simulink model "TheBigOne"  (R2023b)
settings: Solver=FixedStepAuto  StartTime=0.0  StopTime=800.0  RelTol=1e-3
libraries: simulink x5
(part 2 of 2)

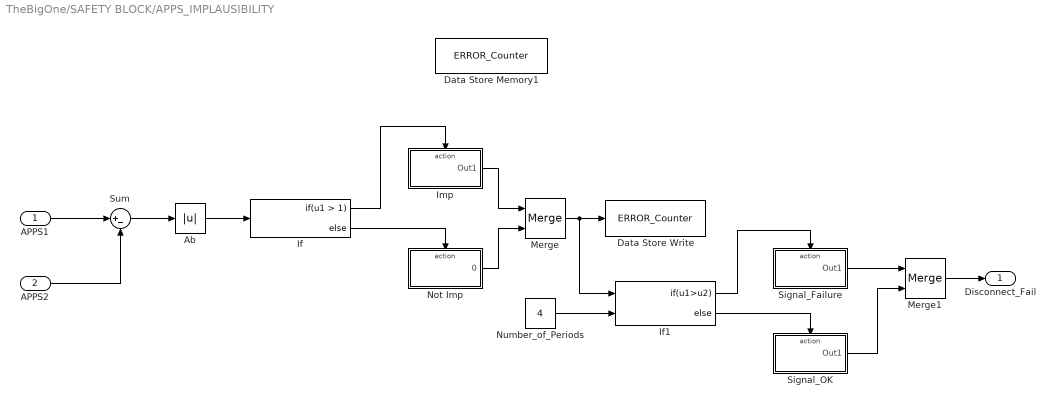
== system TheBigOne/SAFETY BLOCK/APPS_IMPLAUSIBILITY ==
  APPS1 : Inport
  APPS2 : Inport  Port=2
  Ab : Abs  SaturateOnIntegerOverflow=off
  Data Store Memory1 : DataStoreMemory  DataStoreName=ERROR_Counter  ReadBeforeWriteMsg=warning  WriteAfterWriteMsg=warning  WriteAfterReadMsg=warning  ShowAdditionalParam=off
  Data Store Write : DataStoreWrite  DataStoreName=ERROR_Counter  IndexOptions=Index vector (dialog)  Indices=1  OutputSizes=1
  If : If  IfExpression=u1 > 1
  If1 : If  NumInputs=2  IfExpression=u1>u2
  Imp : Subsystem  TreatAsAtomicUnit=on
  Merge : Merge
  Merge1 : Merge
  Not Imp : Subsystem  TreatAsAtomicUnit=on
  Number_of_Periods : Constant  Value=4
  Signal_Failure : Subsystem  TreatAsAtomicUnit=on
  Signal_OK : Subsystem  TreatAsAtomicUnit=on
  Sum : Sum  Inputs=|+-
  Disconnect_Fail : Outport  VectorParamsAs1DForOutWhenUnconnected=off
  wires:
  Number_of_Periods/1 -> If1/2
  Imp/1(Out1) -> Merge/1
  Signal_Failure/1(Out1) -> Merge1/1
  Signal_OK/1(Out1) -> Merge1/2
  Merge1/1 -> Disconnect_Fail/1
  APPS1/1 -> Sum/1
  If/1 -> Imp/Action
  If1/2 -> Signal_OK/Action
  Merge/1 -> Data Store Write/1, If1/1
  If1/1 -> Signal_Failure/Action
  APPS2/1 -> Sum/2
  Ab/1 -> If/1
  If/2 -> Not Imp/Action
  Sum/1 -> Ab/1
  Not Imp/1(0) -> Merge/2

== system TheBigOne/SKIDPAD/RIGIDAXLE ==
  note: TOTAL FAILURE: NO ELIPSE NO INVERTER SPEED
  Throttle_Torque [Nm] : Inport
  Action Port : ActionPort  ActionPortLabel=else
  "Rigid Axle 2024 " : MATLAB Function  TreatAsAtomicUnit=on
  RigidAxle : Constant  Value=4
  Tq_RR_SM4 [Nm] (0,27) : Outport  VectorParamsAs1DForOutWhenUnconnected=off
  Tq_RL_SM4 [Nm] (0,27) : Outport  Port=2  VectorParamsAs1DForOutWhenUnconnected=off
  sensorics_mode : Outport  Port=3
  wires:
  "Rigid Axle 2024 "/1(Motor_Torque_RR) -> Tq_RR_SM4 [Nm] (0,27)/1
  "Rigid Axle 2024 "/2(Motor_Torque_RL) -> Tq_RL_SM4 [Nm] (0,27)/1
  Throttle_Torque [Nm]/1 -> "Rigid Axle 2024 "/1(Throttle_Torque)
  RigidAxle/1 -> sensorics_mode/1

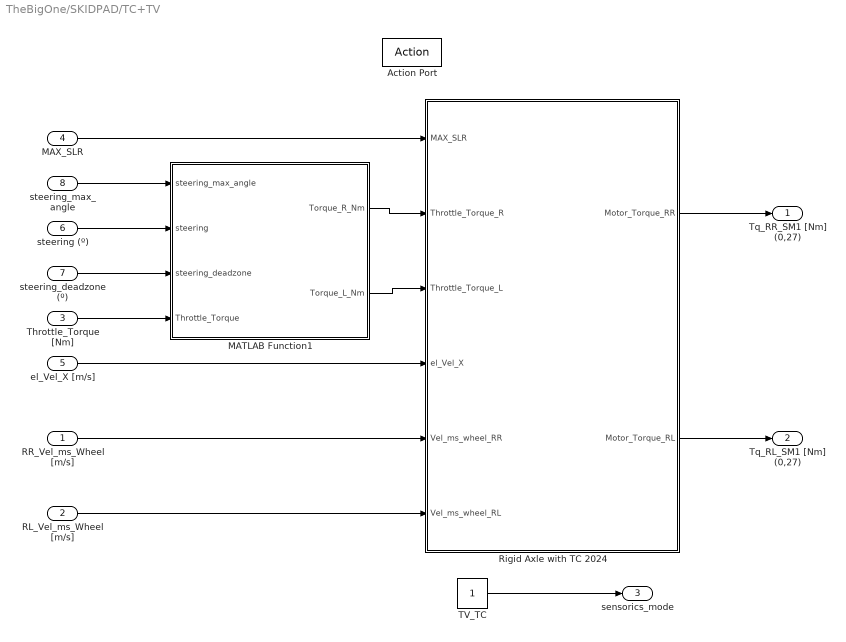
== system TheBigOne/SKIDPAD/TC+TV ==
  RR_Vel_ms_Wheel [m/s] : Inport
  RL_Vel_ms_Wheel [m/s] : Inport  Port=2
  Throttle_Torque [Nm] : Inport  Port=3
  MAX_SLR : Inport  Port=4
  el_Vel_X [m/s] : Inport  Port=5
  steering (º) : Inport  Port=6
  steering_deadzone (º) : Inport  Port=7
  steering_max_angle : Inport  Port=8
  Action Port : ActionPort  ActionPortLabel=if(u1 == 1)
  MATLAB Function1 : MATLAB Function  TreatAsAtomicUnit=on
  "Rigid Axle with TC 2024 " : MATLAB Function  TreatAsAtomicUnit=on
  TV_TC : Constant
  Tq_RR_SM1 [Nm] (0,27) : Outport  VectorParamsAs1DForOutWhenUnconnected=off
  Tq_RL_SM1 [Nm] (0,27) : Outport  Port=2  VectorParamsAs1DForOutWhenUnconnected=off
  sensorics_mode : Outport  Port=3
  wires:
  RR_Vel_ms_Wheel [m/s]/1 -> "Rigid Axle with TC 2024 "/5(Vel_ms_wheel_RR)
  "Rigid Axle with TC 2024 "/1(Motor_Torque_RR) -> Tq_RR_SM1 [Nm] (0,27)/1
  "Rigid Axle with TC 2024 "/2(Motor_Torque_RL) -> Tq_RL_SM1 [Nm] (0,27)/1
  RL_Vel_ms_Wheel [m/s]/1 -> "Rigid Axle with TC 2024 "/6(Vel_ms_wheel_RL)
  Throttle_Torque [Nm]/1 -> MATLAB Function1/4(Throttle_Torque)
  MATLAB Function1/1(Torque_R_Nm) -> "Rigid Axle with TC 2024 "/2(Throttle_Torque_R)
  MAX_SLR/1 -> "Rigid Axle with TC 2024 "/1(MAX_SLR)
  el_Vel_X [m/s]/1 -> "Rigid Axle with TC 2024 "/4(el_Vel_X)
  steering (º)/1 -> MATLAB Function1/2(steering)
  steering_deadzone (º)/1 -> MATLAB Function1/3(steering_deadzone)
  steering_max_angle/1 -> MATLAB Function1/1(steering_max_angle)
  MATLAB Function1/2(Torque_L_Nm) -> "Rigid Axle with TC 2024 "/3(Throttle_Torque_L)
  TV_TC/1 -> sensorics_mode/1

== system TheBigOne/SKIDPAD/TV with TC OFF  ==
  Throttle_Torque [Nm] : Inport
  steering_deadzone : Inport  Port=2
  steering : Inport  Port=3
  steering_max_angle : Inport  Port=4
  Action Port : ActionPort  ActionPortLabel=elseif(u1 <= 3)
  MATLAB Function : MATLAB Function  TreatAsAtomicUnit=on
  SteeringTV : Constant  Value=3
  Tq_RR_SM3 [Nm] (0,27) : Outport  VectorParamsAs1DForOutWhenUnconnected=off
  Tq_RL_SM3 [Nm] (0,27) : Outport  Port=2  VectorParamsAs1DForOutWhenUnconnected=off
  sensorics_mode : Outport  Port=3
  wires:
  Throttle_Torque [Nm]/1 -> MATLAB Function/4(Throttle_Torque)
  steering_deadzone/1 -> MATLAB Function/3(steering_deadzone)
  steering/1 -> MATLAB Function/2(steering)
  steering_max_angle/1 -> MATLAB Function/1(steering_max_angle)
  MATLAB Function/1(Torque_R_Nm) -> Tq_RR_SM3 [Nm] (0,27)/1
  MATLAB Function/2(Torque_L_Nm) -> Tq_RL_SM3 [Nm] (0,27)/1
  SteeringTV/1 -> sensorics_mode/1

== system TheBigOne/TEST_MODE_IN/BYPASS ==
  In1 : Inport
  In2 : Inport  Port=2
  In3 : Inport  Port=3
  In4 : Inport  Port=4
  Action Port : ActionPort  ActionPortLabel=else
  Out1 : Outport  VectorParamsAs1DForOutWhenUnconnected=off
  Out2 : Outport  Port=2  VectorParamsAs1DForOutWhenUnconnected=off
  Out3 : Outport  Port=3  VectorParamsAs1DForOutWhenUnconnected=off
  Out4 : Outport  Port=4  VectorParamsAs1DForOutWhenUnconnected=off
  wires:
  In1/1 -> Out1/1
  In2/1 -> Out2/1
  In3/1 -> Out3/1
  In4/1 -> Out4/1

== system TheBigOne/TEST_MODE_IN/TEST_CONSTANTS ==
  Action Port : ActionPort  ActionPortLabel=if(u1 == 1)
  Constant{,1..3} (4 alike) : Constant  Value=800
  Out1 : Outport  VectorParamsAs1DForOutWhenUnconnected=off
  Out2 : Outport  Port=2  VectorParamsAs1DForOutWhenUnconnected=off
  Out3 : Outport  Port=3  VectorParamsAs1DForOutWhenUnconnected=off
  Out4 : Outport  Port=4  VectorParamsAs1DForOutWhenUnconnected=off
  wires:
  Constant/1 -> Out1/1
  Constant1/1 -> Out2/1
  Constant2/1 -> Out3/1
  Constant3/1 -> Out4/1

== system TheBigOne/Accumulator Power/PowerLimitDetection/LimitReached ==
  Action Port : ActionPort  ActionPortLabel=if(u1 >= 80000)
  Constant : Constant
  "Out " : Outport  VectorParamsAs1DForOutWhenUnconnected=off
  wires:
  Constant/1 -> "Out "/1

== system TheBigOne/Accumulator Power/PowerLimitDetection/OK_OrLatch ==
  IN : Inport
  Action Port : ActionPort  ActionPortLabel=else
  If : If  IfExpression=(u1>0)
  Latched Error : Subsystem  TreatAsAtomicUnit=on
  Merge : Merge
  OK : Subsystem  TreatAsAtomicUnit=on
  Out 1 : Outport  VectorParamsAs1DForOutWhenUnconnected=off
  wires:
  IN/1 -> If/1
  If/1 -> Latched Error/Action
  If/2 -> OK/Action
  Latched Error/1("Out ") -> Merge/1
  OK/1("Out ") -> Merge/2
  Merge/1 -> Out 1/1

== system TheBigOne/ENDURANCE/Velocity cap/If Action Subsystem ==
  Tq_RR : Inport
  Tq_RL : Inport  Port=2
  Action Port : ActionPort  ActionPortLabel=if(u1 > 9)
  Gain : Gain  Gain=0.25
  Gain1 : Gain  Gain=0.25
  TQ_RR : Outport
  TQ_RL : Outport  Port=2
  wires:
  Tq_RL/1 -> Gain1/1
  Gain1/1 -> TQ_RL/1
  Tq_RR/1 -> Gain/1
  Gain/1 -> TQ_RR/1

== system TheBigOne/ENDURANCE/Velocity cap/If Action Subsystem1 ==
  Tq_RR : Inport
  Tq_RL : Inport  Port=2
  Action Port : ActionPort  ActionPortLabel=else
  TQ_RL : Outport
  TQ_RR : Outport  Port=2
  wires:
  Tq_RR/1 -> TQ_RR/1
  Tq_RL/1 -> TQ_RL/1

== system TheBigOne/SAFETY BLOCK/APPS_IMPLAUSIBILITY/Imp ==
  Action Port : ActionPort  ActionPortLabel=if(u1 > 1)
  Add : Sum
  Constant : Constant  OutDataTypeStr=boolean
  Data Store Read : DataStoreRead  DataStoreName=ERROR_Counter  IndexOptions=Index vector (dialog)  Indices=1  OutputSizes=1
  Out1 : Outport  VectorParamsAs1DForOutWhenUnconnected=off
  wires:
  Data Store Read/1 -> Add/1
  Constant/1 -> Add/2
  Add/1 -> Out1/1

== system TheBigOne/SAFETY BLOCK/APPS_IMPLAUSIBILITY/Not Imp ==
  Action Port : ActionPort  ActionPortLabel=else
  Constant : Constant  Value=0  OutDataTypeStr=double
  0 : Outport  VectorParamsAs1DForOutWhenUnconnected=off
  wires:
  Constant/1 -> 0/1  "Boolean"

== system TheBigOne/SAFETY BLOCK/APPS_IMPLAUSIBILITY/Signal_Failure ==
  Action Port : ActionPort  ActionPortLabel=if(u1>u2)
  Constant : Constant
  Out1 : Outport  VectorParamsAs1DForOutWhenUnconnected=off
  wires:
  Constant/1 -> Out1/1

== system TheBigOne/SAFETY BLOCK/APPS_IMPLAUSIBILITY/Signal_OK ==
  Action Port : ActionPort  ActionPortLabel=else
  Constant : Constant  Value=0
  Out1 : Outport  VectorParamsAs1DForOutWhenUnconnected=off
  wires:
  Constant/1 -> Out1/1

== system TheBigOne/Accumulator Power/PowerLimitDetection/OK_OrLatch/Latched Error ==
  Action Port : ActionPort  ActionPortLabel=if((u1>0))
  Constant : Constant
  "Out " : Outport  VectorParamsAs1DForOutWhenUnconnected=off
  wires:
  Constant/1 -> "Out "/1

== system TheBigOne/Accumulator Power/PowerLimitDetection/OK_OrLatch/OK ==
  Action Port : ActionPort  ActionPortLabel=else
  Constant : Constant  Value=0
  "Out " : Outport  VectorParamsAs1DForOutWhenUnconnected=off
  wires:
  Constant/1 -> "Out "/1

== matlab function TheBigOne/Brake_Light ==
  data: BP input; RM input; BL output; PS input; BL_threshold input
function BL = Brake_Light(BP, RM, PS, BL_threshold)
% PS = 0 -> braking
% PS = 1 -> lift
% PS = 2 -> accelerating
% BL_threshold -> BrakePedal percentage to activate BrakeLight
    if ((RM == 5 && PS == 0) || (BP > BL_threshold))
        BL = 1;
        return;
    else
        BL = 0;
        return;
    end
end

== matlab function TheBigOne/Safety ==
  data: Tq_R input; Tq_OK input; Tq_L input; Torque_R output; Torque_L output; W_mot_RR input; W_mot_RL input
function [Torque_R,Torque_L]  = Safety(Tq_R, Tq_OK, Tq_L, W_mot_RR, W_mot_RL)
    if Tq_OK == 1
        Torque_R = Tq_R;
        Torque_L = Tq_L;
        return;
    else
        Torque_R = 0;
        Torque_L = 0;
        return;
    end
end

== matlab function TheBigOne/ACCELERATION/RIGIDAXLE/Rigid Axle 2024  ==
  data: Throttle_Torque input; Motor_Torque_RR output; Motor_Torque_RL output
function [Motor_Torque_RR, Motor_Torque_RL] = RigidAxle_2024(Throttle_Torque)
    
    Motor_Torque_RR = Throttle_Torque;
    Motor_Torque_RL = Throttle_Torque;

end

== matlab function TheBigOne/ACCELERATION/RIGIDAXLE WITH TC/Rigid Axle with TC 2024  ==
  data: MAX_SLR input; Throttle_Torque input; Motor_Torque_RR output; Motor_Torque_RL output; el_Vel_X input; Max_Vel_ms_Wheel input
function [Motor_Torque_RR, Motor_Torque_RL] = RigidAxle_TC_2024(MAX_SLR, Throttle_Torque, el_Vel_X, Max_Vel_ms_Wheel)    
    persistent correction
    if isempty(correction)
        correction = 0;
    end
if (el_Vel_X < 0.5 || Max_Vel_ms_Wheel < 0.5)
    correction = 0;
    Motor_Torque_RR = Throttle_Torque;
    Motor_Torque_RL = Throttle_Torque;
    return;
else

% SLIP RATIO CALCULATIONS
    % calculate slip ratio
    if(el_Vel_X == 0 ||Max_Vel_ms_Wheel == 0)
        SLR = 1;
    else
    SLR = (Max_Vel_ms_Wheel / el_Vel_X);
    end
% CHECK FOR EXCESIVE SLIPPING
    % SLIP RATIO LESSER THAN MAXIMUM SLIP RATIO => apply max torque times throttle factor
        if(SLR < MAX_SLR)
            Motor_Torque_RR = Throttle_Torque; 
            Motor_Torque_RL = Throttle_Torque;
            correction = 0; %set correction to 0 as tyre is not slipping
            return;
        else
        % TYRE SLIPPING => TC INTERVENES
            % LOOK FOR THE PREVIOUS CORRECTION [Nm]
            if (correction == 0) % NOT SLIPPING PREVIOUSLY
                correction = 1; % [INTERVAL TO BE DETERMINED] set the correction to the torque we want to substract
                Motor_Torque_RR = Throttle_Torque - (1/33*correction^2+1/33*correction); % substract the correction from the torque to apply
                Motor_Torque_RL = Throttle_Torque - (1/33*correction^2+1/33*correction);
                return;
            else % TYRE SLIPPING PREVIOUSLY
                correction = correction + 1; % [INTERVAL TO BE DETERMINED] set the correction to the torque we want to substract + previous corrections
                Motor_Torque_RR = Throttle_Torque - (1/33*correction^2+1/33*correction); % substract the correction from the torque to apply
                Motor_Torque_RL = Throttle_Torque - (1/33*correction^2+1/33*correction);
                return;
            end
        end
end
end

== matlab function TheBigOne/ENDURANCE/RIGIDAXLE WITH TC/Rigid Axle with TC 2024  ==
  data: MAX_SLR input; Throttle_Torque input; Motor_Torque_RR output; Motor_Torque_RL output; el_Vel_X input; Max_Vel_ms_Wheel input
function [Motor_Torque_RR, Motor_Torque_RL] = RigidAxle_TC_2024(MAX_SLR, Throttle_Torque, el_Vel_X, Max_Vel_ms_Wheel)    
    persistent correction
    if isempty(correction)
        correction = 0;
    end
if (el_Vel_X < 0.5 || Max_Vel_ms_Wheel < 0.5)
    Motor_Torque_RR = Throttle_Torque;
    Motor_Torque_RL = Throttle_Torque;
    return;
else

% SLIP RATIO CALCULATIONS
    % calculate slip ratio
    if(el_Vel_X == 0 ||Max_Vel_ms_Wheel == 0)
        SLR = 1;
    else
    SLR = (Max_Vel_ms_Wheel / el_Vel_X);
    end
% CHECK FOR EXCESIVE SLIPPING
    % SLIP RATIO LESSER THAN MAXIMUM SLIP RATIO => apply max torque times throttle factor
        if(SLR < MAX_SLR)
            Motor_Torque_RR = Throttle_Torque; 
            Motor_Torque_RL = Throttle_Torque;
            correction = 0; %set correction to 0 as tyre is not slipping
            return;
        else
        % TYRE SLIPPING => TC INTERVENES
            % LOOK FOR THE PREVIOUS CORRECTION [Nm]
            if (correction == 0) % NOT SLIPPING PREVIOUSLY
                correction = 1; % [INTERVAL TO BE DETERMINED] set the correction to the torque we want to substract
                Motor_Torque_RR = Throttle_Torque - (1/33*correction^2+1/33*correction); % substract the correction from the torque to apply
                Motor_Torque_RL = Throttle_Torque - (1/33*correction^2+1/33*correction);
                return;
            else % TYRE SLIPPING PREVIOUSLY
                correction = correction + 1; % [INTERVAL TO BE DETERMINED] set the correction to the torque we want to substract + previous corrections
                Motor_Torque_RR = Throttle_Torque - (1/33*correction^2+1/33*correction); % substract the correction from the torque to apply
                Motor_Torque_RL = Throttle_Torque - (1/33*correction^2+1/33*correction);
                return;
            end
        end
end
end

== matlab function TheBigOne/ENDURANCE/TC+TV/TC 2024 ==
  data: MAX_SLR input; Throttle_Torque_R input; Throttle_Torque_L input; Motor_Torque_RR output; Motor_Torque_RL output; el_Vel_X input; Vel_ms_wheel_RR input; Vel_ms_wheel_RL input
function [Motor_Torque_RR, Motor_Torque_RL] = TC_2024(MAX_SLR,Throttle_Torque_R, Throttle_Torque_L, el_Vel_X, Vel_ms_wheel_RR, Vel_ms_wheel_RL)
    persistent correction
    if isempty(correction)
        correction = 0;
    end
if (el_Vel_X < 0.5 || Vel_ms_wheel_RR < 0.5 || Vel_ms_wheel_RL < 0.5)
    Motor_Torque_RR = Throttle_Torque_R;
    Motor_Torque_RL = Throttle_Torque_L;
    return;
else

% SLIP RATIO CALCULATIONS
    % calculate slip ratio
    if(el_Vel_X == 0 || Vel_ms_wheel_RR == 0)
        SLR_RR = 1;
    else
    SLR_RR = (Vel_ms_wheel_RR / el_Vel_X);
    end
    if(el_Vel_X == 0 || Vel_ms_wheel_RL == 0)
        SLR_RL = 1;
    else
    SLR_RL = (Vel_ms_wheel_RL / el_Vel_X);
    end


% SLIP RATIO CALCULATIONS
    % calculate slip ratio
    SLR = max(SLR_RR, SLR_RL);

% CHECK FOR EXCESIVE SLIPPING
    % SLIP RATIO LESSER THAN MAXIMUM SLIP RATIO => apply max torque times throttle factor
        if(SLR < MAX_SLR)
            Motor_Torque_RR = Throttle_Torque_R; 
            Motor_Torque_RL = Throttle_Torque_L;
            correction = 0; %set correction to 0 as tyre is not slipping
            return;
        else
        % TYRE SLIPPING => TC INTERVENES
            % LOOK FOR THE PREVIOUS CORRECTION [Nm]
            if (correction == 0) % NOT SLIPPING PREVIOUSLY
                correction = 1; % [INTERVAL TO BE DETERMINED] set the correction to the torque we want to substract
                Motor_Torque_RR = Throttle_Torque_R - (1/33*correction^2+1/33*correction); % substract the correction from the torque to apply
                Motor_Torque_RL = Throttle_Torque_L - (1/33*correction^2+1/33*correction);
                return;
            else % TYRE SLIPPING PREVIOUSLY
                correction = correction + 1; % [INTERVAL TO BE DETERMINED] set the correction to the torque we want to substract + previous corrections
                Motor_Torque_RR = Throttle_Torque_R - (1/33*correction^2+1/33*correction); % substract the correction from the torque to apply
                Motor_Torque_RL = Throttle_Torque_L - (1/33*correction^2+1/33*correction);
                return;
            end
        end
end
end

== matlab function TheBigOne/ACCELERATION/Torque demanded by the driver ==
  data: Throttle_Torque output; AP input; pedal_sat_down input; pedal_sat_up input; max_torque input
function Throttle_Torque  = TT(AP, pedal_sat_down, pedal_sat_up, max_torque)
    if AP <= pedal_sat_down %establish the lower deadzone for the throttle pedal
        Throttle_Response = 0;

    elseif AP >= pedal_sat_up %establish the higher deadzone for the throttle pedal
        Throttle_Response = 1;

    else
        Throttle_Response = ((AP - pedal_sat_down) / (pedal_sat_up - pedal_sat_down)); %evaluate for given input
    end
    Throttle_Torque = Throttle_Response * max_torque; % set torque to max output times pedal factor
end

== matlab function TheBigOne/InverterL_Temp_Limitation ==
  data: Current_in input; Aggressive_Factor input; Max_Temp input; Current_out output; Tolerance input; Inv_Temp input; Change_Factor input
function Current_out = Inv_Temp(Current_in, Aggressive_Factor, Max_Temp, Tolerance, Inv_Temp, Change_Factor)
%% Initializing internal variables
% If they have not been defined yet, initiate them

    % Last_Temp (ºC) -> Inv_Temp of the last iteration
    persistent Last_Temp
    if isempty(Last_Temp)
        Last_Temp = 0;
    end

    % Aggressive Factor Value (%) -> Factor of Current reduction. Changes
    % every iteration due to counters, but can be reset if the Inv_Temp is
    % acceptable
    persistent AF_Value
    if isempty(AF_Value)
        AF_Value = Aggressive_Factor;
    end

    % Times_Incremented -> Counter of the Temp_Change higher than Tolerance
    persistent Times_Incremented
    if isempty(Times_Incremented)
        Times_Incremented = 1;
    end

    % Times_Decremented -> Counter of the Temp_Change lower than -Tolerance
    persistent Times_Decremented
    if isempty(Times_Decremented)
        Times_Decremented = 1;
    end

%% Derivative
    % Compute the Temperature difference between the last temp and the
    % actual one
Temp_Change = Inv_Temp - Last_Temp;

%% Temperature Control Logic
    
    if (Temp_Change > Tolerance)
        % Temperature is increasing beyond Tolerance, limit the Current
        % more aggressively to reduce the Inv_Temp
        New_Current = Current_in * (1 - (AF_Value * Temp_Change / 100));
        % Increase the Aggresive Factor for the next iteration and sum 1 to
        % the Increment counter
        AF_Value = AF_Value + (Change_Factor * Times_Incremented);
        Times_Incremented = Times_Incremented + 1;
        Times_Decremented = 1;

    elseif (Temp_Change < -Tolerance)
        % Temperature is cooling down beyond Tolerance, allow to normalize
        % the Current (then the temperature rises)
        New_Current = Current_in * (1 - (AF_Value * Temp_Change / 100));
        % Decrease the Aggressive Factor for the next iteration and sum 1
        % to the Decrement counter
        AF_Value = AF_Value - (Change_Factor * Times_Decremented);
        Times_Incremented = 1;
        Times_Decremented = Times_Decremented + 1;

    else
        % Temperature is stable (within Tolerance), gradually reduce Current
        New_Current = Current_in * (1 - AF_Value / 10);
        % Reset both counters
        Times_Incremented = 1;
        Times_Decremented = 1;

    end
%% Compare the Actual Current with the New Current

    if (((New_Current > Current_in) && (Current_in >= 0)) || ((New_Current < Current_in) && (Current_in < 0)))
        % Ensure the New_Current does not exceed the input current when accelerating
        % If regen, then the New_Current cannot be lower than the Current_in, it
        % has to be higher (they are both negative)
        New_Current = Current_in;

    elseif (sign(New_Current) ~= sign(Current_in))
        % If it was demanding a positive current, but New_Current is
        % negative, just output 0 (so we do not regenerate when we don't
        % want). Same for the inverse case
        New_Current = 0;
        
    end

%% Output values

    if (Inv_Temp > Max_Temp)
        % If the Inv_Temp is higher than the Maximum_Temp selected, limit
        % the Current with the calculated one
        Current_out = New_Current;

    else
        % If the Inv_Temp is acceptable, maintain the current demanded and
        % do not apply the calculated Aggresive Factor Value
        Current_out = Current_in;
        AF_Value = Aggressive_Factor;

    end
% Update the last known Temperature
Last_Temp = Inv_Temp;
end

== matlab function TheBigOne/ENDURANCE/Torque/state ==
  data: AP input; AP_sat_down input; state output; AP_sat_mid input
function state = Pedal_State(AP, AP_sat_down, AP_sat_mid)
% state = 0 -> braking
% state = 1 -> lift
% state = 2 -> accelerating
state = 1;
if AP < AP_sat_down
    state = 0;
    return;
end
if AP >= AP_sat_down && AP <= AP_sat_mid
    state = 1;
    return;
end
if AP > AP_sat_mid
    state = 2;
    return;
end
end

== matlab function TheBigOne/AUTOX1/TC+TV/Rigid Axle with TC 2024  ==
  data: MAX_SLR input; Throttle_Torque_R input; Throttle_Torque_L input; Motor_Torque_RR output; Motor_Torque_RL output; el_Vel_X input; Vel_ms_wheel_RR input; Vel_ms_wheel_RL input
function [Motor_Torque_RR, Motor_Torque_RL] = TC_2024(MAX_SLR,Throttle_Torque_R, Throttle_Torque_L, el_Vel_X, Vel_ms_wheel_RR, Vel_ms_wheel_RL)
    persistent correction
    if isempty(correction)
        correction = 0;
    end
if (el_Vel_X < 0.5 || Vel_ms_wheel_RR < 0.5 || Vel_ms_wheel_RL < 0.5)
    correction = 0;
    Motor_Torque_RR = Throttle_Torque_R;
    Motor_Torque_RL = Throttle_Torque_L;
    return;
else
    
% SLIP RATIO CALCULATIONS
    % calculate slip ratio
    if(el_Vel_X == 0 || Vel_ms_wheel_RR == 0)
        SLR_RR = 1;
    else
    SLR_RR = (Vel_ms_wheel_RR / el_Vel_X);
    end
    if(el_Vel_X == 0 || Vel_ms_wheel_RL == 0)
        SLR_RL = 1;
    else
    SLR_RL = (Vel_ms_wheel_RL / el_Vel_X);
    end


% SLIP RATIO CALCULATIONS
    % calculate slip ratio
    SLR = max(SLR_RR, SLR_RL);

% CHECK FOR EXCESIVE SLIPPING
    % SLIP RATIO LESSER THAN MAXIMUM SLIP RATIO => apply max torque times throttle factor
        if(SLR < MAX_SLR)
            Motor_Torque_RR = Throttle_Torque_R; 
            Motor_Torque_RL = Throttle_Torque_L;
            correction = 0; %set correction to 0 as tyre is not slipping
            return;
        else
        % TYRE SLIPPING => TC INTERVENES
            % LOOK FOR THE PREVIOUS CORRECTION [Nm]
            if (correction == 0) % NOT SLIPPING PREVIOUSLY
                correction = 1; % [INTERVAL TO BE DETERMINED] set the correction to the torque we want to substract
                Motor_Torque_RR = Throttle_Torque_R - (1/33*correction^2+1/33*correction); % substract the correction from the torque to apply
                Motor_Torque_RL = Throttle_Torque_L - (1/33*correction^2+1/33*correction);
                return;
            else % TYRE SLIPPING PREVIOUSLY
                correction = correction + 1; % [INTERVAL TO BE DETERMINED] set the correction to the torque we want to substract + previous corrections
                Motor_Torque_RR = Throttle_Torque_R - (1/33*correction^2+1/33*correction); % substract the correction from the torque to apply
                Motor_Torque_RL = Throttle_Torque_L - (1/33*correction^2+1/33*correction);
                return;
            end
        end
end
end

== matlab function TheBigOne/SKIDPAD/TV with TC OFF /MATLAB Function ==
  data: steering_max_angle input; Torque_R_Nm output; Torque_L_Nm output; steering input; steering_deadzone input; Throttle_Torque input
function [Torque_R_Nm, Torque_L_Nm] = TV(steering_max_angle, steering, steering_deadzone, Throttle_Torque)

if abs(steering) <= steering_deadzone % add steering deadzone (º)
    Torque_L_Nm = Throttle_Torque;
    Torque_R_Nm = Throttle_Torque;
    return;
end
d = (abs(steering) - steering_deadzone)/(steering_max_angle - steering_deadzone) * Throttle_Torque; %evaluate delta torque for given steering angle
if d > Throttle_Torque
     d = Throttle_Torque; %force torque to be positive to avoid balance issues
end
if steering < -steering_deadzone %if steering left, apply full torque to the emotor on the outside
    Torque_L_Nm = Throttle_Torque-d;
    Torque_R_Nm = Throttle_Torque;
    return;
else
%opposite case
Torque_L_Nm = Throttle_Torque;
Torque_R_Nm = Throttle_Torque-d;
return;
end
end

== matlab function TheBigOne/WORKSHOP/Torque demanded by the driver ==
  data: Throttle_Torque output; AP input; pedal_sat_down input; pedal_sat_up input; max_torque input; max_wheel_w input
function Throttle_Torque  = TT(AP, pedal_sat_down, pedal_sat_up, max_torque, max_wheel_w)
max_torque = max_torque / 9; % Max Tq = 3Nm
    if AP <= pedal_sat_down || max_wheel_w > 5 % establish the lower deadzone for the throttle pedal
        Throttle_Response = 0;

    elseif AP >= pedal_sat_up % establish the higher deadzone for the throttle pedal
        Throttle_Response = 1;

    else
        Throttle_Response = ((AP - pedal_sat_down) / (pedal_sat_up - pedal_sat_down)); %evaluate for given input
    end
    Throttle_Torque = Throttle_Response * max_torque; % set torque to max output times pedal factor
end

== matlab function TheBigOne/InverterR_Temp_Limitation ==
  data: Current_in input; Aggressive_Factor input; Max_Temp input; Current_out output; Tolerance input; Inv_Temp input; Change_Factor input
function Current_out = Inv_Temp(Current_in, Aggressive_Factor, Max_Temp, Tolerance, Inv_Temp, Change_Factor)
%% Initializing internal variables
% If they have not been defined yet, initiate them

    % Last_Temp (ºC) -> Inv_Temp of the last iteration
    persistent Last_Temp
    if isempty(Last_Temp)
        Last_Temp = 0;
    end

    % Aggressive Factor Value (%) -> Factor of Current reduction. Changes
    % every iteration due to counters, but can be reset if the Inv_Temp is
    % acceptable
    persistent AF_Value
    if isempty(AF_Value)
        AF_Value = Aggressive_Factor;
    end

    % Times_Incremented -> Counter of the Temp_Change higher than Tolerance
    persistent Times_Incremented
    if isempty(Times_Incremented)
        Times_Incremented = 1;
    end

    % Times_Decremented -> Counter of the Temp_Change lower than -Tolerance
    persistent Times_Decremented
    if isempty(Times_Decremented)
        Times_Decremented = 1;
    end

%% Derivative
    % Compute the Temperature difference between the last temp and the
    % actual one
Temp_Change = Inv_Temp - Last_Temp;

%% Temperature Control Logic
    
    if (Temp_Change > Tolerance)
        % Temperature is increasing beyond Tolerance, limit the Current
        % more aggressively to reduce the Inv_Temp
        New_Current = Current_in * (1 - (AF_Value * Temp_Change / 100));
        % Increase the Aggresive Factor for the next iteration and sum 1 to
        % the Increment counter
        AF_Value = AF_Value + (Change_Factor * Times_Incremented);
        Times_Incremented = Times_Incremented + 1;
        Times_Decremented = 1;

    elseif (Temp_Change < -Tolerance)
        % Temperature is cooling down beyond Tolerance, allow to normalize
        % the Current (then the temperature rises)
        New_Current = Current_in * (1 - (AF_Value * Temp_Change / 100));
        % Decrease the Aggressive Factor for the next iteration and sum 1
        % to the Decrement counter
        AF_Value = AF_Value - (Change_Factor * Times_Decremented);
        Times_Incremented = 1;
        Times_Decremented = Times_Decremented + 1;

    else
        % Temperature is stable (within Tolerance), gradually reduce Current
        New_Current = Current_in * (1 - AF_Value / 10);
        % Reset both counters
        Times_Incremented = 1;
        Times_Decremented = 1;

    end
%% Compare the Actual Current with the New Current

    if (((New_Current > Current_in) && (Current_in >= 0)) || ((New_Current < Current_in) && (Current_in < 0)))
        % Ensure the New_Current does not exceed the input current when accelerating
        % If regen, then the New_Current cannot be lower than the Current_in, it
        % has to be higher (they are both negative)
        New_Current = Current_in;

    elseif (sign(New_Current) ~= sign(Current_in))
        % If it was demanding a positive current, but New_Current is
        % negative, just output 0 (so we do not regenerate when we don't
        % want). Same for the inverse case
        New_Current = 0;
        
    end

%% Output values

    if (Inv_Temp > Max_Temp)
        % If the Inv_Temp is higher than the Maximum_Temp selected, limit
        % the Current with the calculated one
        Current_out = New_Current;

    else
        % If the Inv_Temp is acceptable, maintain the current demanded and
        % do not apply the calculated Aggresive Factor Value
        Current_out = Current_in;
        AF_Value = Aggressive_Factor;

    end
% Update the last known Temperature
Last_Temp = Inv_Temp;
end

== matlab function TheBigOne/ENDURANCE/Torque/enable regen ==
  data: regen_en output; SOC input; max_SOC input; current input; voltage input; W_RR input; W_RL input; max_regen_torque_RR output; max_regen_torque_RL output
function [regen_en, max_regen_torque_RR, max_regen_torque_RL] = regen(SOC, max_SOC, current, voltage, W_RR, W_RL)
    max_regen_torque_RR = 0;
    max_regen_torque_RL = 0;
    regen_en = 0;
    if SOC < max_SOC && min(W_RR, W_RL) > 33 %If W is lower (< 2.4 km/h), do not regen to avoid going backwards
        regen_en = 1;
    end
    if SOC >= max_SOC
        regen_en = 0;
    end
    if regen_en == 1
        max_regen_torque_RR = min(current*voltage/W_RR, 27);
        max_regen_torque_RL = min(current*voltage/W_RL, 27);
    end
end

== matlab function TheBigOne/ENDURANCE/Torque/Torque demanded by the driver ==
  data: max_regen_torque input; regen_en input; state input; AP input; AP_sat_down input; AP_sat_mid input; tq_RR output; tq_RL output; max_torque input
function [tq_RR, tq_RL] = torque(max_regen_torque, regen_en, state, AP, AP_sat_down, AP_sat_mid, max_torque)
% state = 0 -> braking
% state = 1 -> lift
% state = 2 -> accelerating
    tq_RR = 0;
    tq_RL = 0;
    if state == 0
        if regen_en == 1
        tq_RR = AP * (max_regen_torque/AP_sat_down) - max_regen_torque;
        tq_RL = tq_RR;
        else
            tq_RR = 0;
            tq_RL = 0;
        end
    end
    if state == 1
        tq_RR = 0;
        tq_RL = 0;
    end
    if state == 2
        tq_RR = max_torque * ((AP-AP_sat_mid) / (1 - AP_sat_mid));
        tq_RL = tq_RR;
    end
end

== matlab function TheBigOne/AUTOX1/RIGIDAXLE/Rigid Axle 2024  ==
  data: Throttle_Torque input; Motor_Torque_RR output; Motor_Torque_RL output
function [Motor_Torque_RR, Motor_Torque_RL] = RigidAxle_2024(Throttle_Torque)
    
    Motor_Torque_RR = Throttle_Torque;
    Motor_Torque_RL = Throttle_Torque;

end

== matlab function TheBigOne/ENDURANCE/RIGIDAXLE/Rigid Axle 2024  ==
  data: Throttle_Torque input; Motor_Torque_RR output; Motor_Torque_RL output
function [Motor_Torque_RR, Motor_Torque_RL] = RigidAxle_2024(Throttle_Torque)
    
    Motor_Torque_RR = Throttle_Torque;
    Motor_Torque_RL = Throttle_Torque;

end

== matlab function TheBigOne/MotorL_Temp_Limitation ==
  data: Current_in input; Aggressive_Factor input; Max_Temp input; Current_out output; Tolerance input; Mot_Temp input; Change_Factor input
function Current_out = Mot_Temp(Current_in, Aggressive_Factor, Max_Temp, Tolerance, Mot_Temp, Change_Factor)
%% Initializing internal variables
% If they have not been defined yet, initiate them

    % Last_Temp (ºC) -> Mot_Temp of the last iteration
    persistent Last_Temp
    if isempty(Last_Temp)
        Last_Temp = 0;
    end

    % Aggressive Factor Value (%) -> Factor of Current reduction. Changes
    % every iteration due to counters, but can be reset if the Mot_Temp is
    % acceptable
    persistent AF_Value
    if isempty(AF_Value)
        AF_Value = Aggressive_Factor;
    end

    % Times_Incremented -> Counter of the Temp_Change higher than Tolerance
    persistent Times_Incremented
    if isempty(Times_Incremented)
        Times_Incremented = 1;
    end

    % Times_Decremented -> Counter of the Temp_Change lower than -Tolerance
    persistent Times_Decremented
    if isempty(Times_Decremented)
        Times_Decremented = 1;
    end

%% Derivative
    % Compute the Temperature difference between the last temp and the
    % actual one
Temp_Change = Mot_Temp - Last_Temp;

%% Temperature Control Logic
    
    if (Temp_Change > Tolerance)
        % Temperature is increasing beyond Tolerance, limit the Current
        % more aggressively to reduce the Mot_Temp
        New_Current = Current_in * (1 - (AF_Value * Temp_Change / 100));
        % Increase the Aggresive Factor for the next iteration and sum 1 to
        % the Increment counter
        AF_Value = AF_Value + (Change_Factor * Times_Incremented);
        Times_Incremented = Times_Incremented + 1;
        Times_Decremented = 1;

    elseif (Temp_Change < -Tolerance)
        % Temperature is cooling down beyond Tolerance, allow to normalize
        % the Current (then the temperature rises)
        New_Current = Current_in * (1 - (AF_Value * Temp_Change / 100));
        % Decrease the Aggressive Factor for the next iteration and sum 1
        % to the Decrement counter
        AF_Value = AF_Value - (Change_Factor * Times_Decremented);
        Times_Incremented = 1;
        Times_Decremented = Times_Decremented + 1;

    else
        % Temperature is stable (within Tolerance), gradually reduce Current
        New_Current = Current_in * (1 - AF_Value / 10);
        % Reset both counters
        Times_Incremented = 1;
        Times_Decremented = 1;

    end
%% Compare the Actual Current with the New Current

    if (((New_Current > Current_in) && (Current_in >= 0)) || ((New_Current < Current_in) && (Current_in < 0)))
        % Ensure the New_Current does not exceed the input current when accelerating
        % If regen, then the New_Current cannot be lower than the Current_in, it
        % has to be higher (they are both negative)
        New_Current = Current_in;

    elseif (sign(New_Current) ~= sign(Current_in))
        % If it was demanding a positive current, but New_Current is
        % negative, just output 0 (so we do not regenerate when we don't
        % want). Same for the inverse case
        New_Current = 0;
        
    end

%% Output values

    if (Mot_Temp > Max_Temp)
        % If the Mot_Temp is higher than the Maximum_Temp selected, limit
        % the Current with the calculated one
        Current_out = New_Current;

    else
        % If the Mot_Temp is acceptable, maintain the current demanded and
        % do not apply the calculated Aggresive Factor Value
        Current_out = Current_in;
        AF_Value = Aggressive_Factor;

    end
% Update the last known Temperature
Last_Temp = Mot_Temp;
end

== matlab function TheBigOne/SKIDPAD/RIGIDAXLE/Rigid Axle 2024  ==
  data: Throttle_Torque input; Motor_Torque_RR output; Motor_Torque_RL output
function [Motor_Torque_RR, Motor_Torque_RL] = RigidAxle_2024(Throttle_Torque)
    
    Motor_Torque_RR = Throttle_Torque;
    Motor_Torque_RL = Throttle_Torque;

end

== matlab function TheBigOne/MotorR_Temp_Limitation ==
  data: Current_in input; Aggressive_Factor input; Max_Temp input; Current_out output; Tolerance input; Mot_Temp input; Change_Factor input
function Current_out = Mot_Temp(Current_in, Aggressive_Factor, Max_Temp, Tolerance, Mot_Temp, Change_Factor)
%% Initializing internal variables
% If they have not been defined yet, initiate them

    % Last_Temp (ºC) -> Mot_Temp of the last iteration
    persistent Last_Temp
    if isempty(Last_Temp)
        Last_Temp = 0;
    end

    % Aggressive Factor Value (%) -> Factor of Current reduction. Changes
    % every iteration due to counters, but can be reset if the Mot_Temp is
    % acceptable
    persistent AF_Value
    if isempty(AF_Value)
        AF_Value = Aggressive_Factor;
    end

    % Times_Incremented -> Counter of the Temp_Change higher than Tolerance
    persistent Times_Incremented
    if isempty(Times_Incremented)
        Times_Incremented = 1;
    end

    % Times_Decremented -> Counter of the Temp_Change lower than -Tolerance
    persistent Times_Decremented
    if isempty(Times_Decremented)
        Times_Decremented = 1;
    end

%% Derivative
    % Compute the Temperature difference between the last temp and the
    % actual one
Temp_Change = Mot_Temp - Last_Temp;

%% Temperature Control Logic
    
    if (Temp_Change > Tolerance)
        % Temperature is increasing beyond Tolerance, limit the Current
        % more aggressively to reduce the Mot_Temp
        New_Current = Current_in * (1 - (AF_Value * Temp_Change / 100));
        % Increase the Aggresive Factor for the next iteration and sum 1 to
        % the Increment counter
        AF_Value = AF_Value + (Change_Factor * Times_Incremented);
        Times_Incremented = Times_Incremented + 1;
        Times_Decremented = 1;

    elseif (Temp_Change < -Tolerance)
        % Temperature is cooling down beyond Tolerance, allow to normalize
        % the Current (then the temperature rises)
        New_Current = Current_in * (1 - (AF_Value * Temp_Change / 100));
        % Decrease the Aggressive Factor for the next iteration and sum 1
        % to the Decrement counter
        AF_Value = AF_Value - (Change_Factor * Times_Decremented);
        Times_Incremented = 1;
        Times_Decremented = Times_Decremented + 1;

    else
        % Temperature is stable (within Tolerance), gradually reduce Current
        New_Current = Current_in * (1 - AF_Value / 10);
        % Reset both counters
        Times_Incremented = 1;
        Times_Decremented = 1;

    end
%% Compare the Actual Current with the New Current

    if (((New_Current > Current_in) && (Current_in >= 0)) || ((New_Current < Current_in) && (Current_in < 0)))
        % Ensure the New_Current does not exceed the input current when accelerating
        % If regen, then the New_Current cannot be lower than the Current_in, it
        % has to be higher (they are both negative)
        New_Current = Current_in;

    elseif (sign(New_Current) ~= sign(Current_in))
        % If it was demanding a positive current, but New_Current is
        % negative, just output 0 (so we do not regenerate when we don't
        % want). Same for the inverse case
        New_Current = 0;
        
    end

%% Output values

    if (Mot_Temp > Max_Temp)
        % If the Mot_Temp is higher than the Maximum_Temp selected, limit
        % the Current with the calculated one
        Current_out = New_Current;

    else
        % If the Mot_Temp is acceptable, maintain the current demanded and
        % do not apply the calculated Aggresive Factor Value
        Current_out = Current_in;
        AF_Value = Aggressive_Factor;

    end
% Update the last known Temperature
Last_Temp = Mot_Temp;
end

== matlab function TheBigOne/SKIDPAD/TC+TV/MATLAB Function1 ==
  data: steering_max_angle input; Torque_R_Nm output; Torque_L_Nm output; steering input; steering_deadzone input; Throttle_Torque input
function [Torque_R_Nm, Torque_L_Nm] = TV(steering_max_angle, steering, steering_deadzone, Throttle_Torque)

if abs(steering) <= steering_deadzone % add steering deadzone (º)
    Torque_L_Nm = Throttle_Torque;
    Torque_R_Nm = Throttle_Torque;
    return;
end
d = (abs(steering) - steering_deadzone)/(steering_max_angle - steering_deadzone) * Throttle_Torque; %evaluate delta torque for given steering angle
if d > Throttle_Torque
     d = Throttle_Torque; %force torque to be positive to avoid balance issues
end
if steering < -steering_deadzone %if steering left, apply full torque to the emotor on the outside
    Torque_L_Nm = Throttle_Torque-d;
    Torque_R_Nm = Throttle_Torque;
    return;
else
%opposite case
Torque_L_Nm = Throttle_Torque;
Torque_R_Nm = Throttle_Torque-d;
return;
end
end

== matlab function TheBigOne/AUTOX1/RIGIDAXLE WITH TC/Rigid Axle with TC 2024  ==
  data: MAX_SLR input; Throttle_Torque input; Motor_Torque_RR output; Motor_Torque_RL output; el_Vel_X input; Max_Vel_ms_Wheel input
function [Motor_Torque_RR, Motor_Torque_RL] = RigidAxle_TC_2024(MAX_SLR, Throttle_Torque, el_Vel_X, Max_Vel_ms_Wheel)    
    persistent correction
    if isempty(correction)
        correction = 0;
    end
if (el_Vel_X < 0.5 || Max_Vel_ms_Wheel < 0.5)
    correction = 0;
    Motor_Torque_RR = Throttle_Torque;
    Motor_Torque_RL = Throttle_Torque;
    return;
else

% SLIP RATIO CALCULATIONS
    % calculate slip ratio
    if(el_Vel_X == 0 ||Max_Vel_ms_Wheel == 0)
        SLR = 1;
    else
    SLR = (Max_Vel_ms_Wheel / el_Vel_X);
    end
% CHECK FOR EXCESIVE SLIPPING
    % SLIP RATIO LESSER THAN MAXIMUM SLIP RATIO => apply max torque times throttle factor
        if(SLR < MAX_SLR)
            Motor_Torque_RR = Throttle_Torque; 
            Motor_Torque_RL = Throttle_Torque;
            correction = 0; %set correction to 0 as tyre is not slipping
            return;
        else
        % TYRE SLIPPING => TC INTERVENES
            % LOOK FOR THE PREVIOUS CORRECTION [Nm]
            if (correction == 0) % NOT SLIPPING PREVIOUSLY
                correction = 1; % [INTERVAL TO BE DETERMINED] set the correction to the torque we want to substract
                Motor_Torque_RR = Throttle_Torque - (1/33*correction^2+1/33*correction); % substract the correction from the torque to apply
                Motor_Torque_RL = Throttle_Torque - (1/33*correction^2+1/33*correction);
                return;
            else % TYRE SLIPPING PREVIOUSLY
                correction = correction + 1; % [INTERVAL TO BE DETERMINED] set the correction to the torque we want to substract + previous corrections
                Motor_Torque_RR = Throttle_Torque - (1/33*correction^2+1/33*correction); % substract the correction from the torque to apply
                Motor_Torque_RL = Throttle_Torque - (1/33*correction^2+1/33*correction);
                return;
            end
        end
end
end

== matlab function TheBigOne/ENDURANCE/TC+TV/MATLAB Function1 ==
  data: steering_max_angle input; Torque_R_Nm output; Torque_L_Nm output; steering input; steering_deadzone input; Throttle_Torque input; regen_en input
function [Torque_R_Nm, Torque_L_Nm] = TV(steering_max_angle, steering, steering_deadzone, Throttle_Torque, regen_en)

if abs(steering) <= steering_deadzone % add steering deadzone (º)
    Torque_L_Nm = Throttle_Torque;
    Torque_R_Nm = Throttle_Torque;
    return;
end
d = (abs(steering) - steering_deadzone)/(steering_max_angle - steering_deadzone) * Throttle_Torque; %evaluate delta torque for given steering angle

if regen_en == 0 && d > Throttle_Torque
     d = Throttle_Torque; %force torque to be positive to avoid balance issues
end
if steering < -steering_deadzone %if steering left, apply full torque to the emotor on the inside
    Torque_L_Nm = Throttle_Torque;
    Torque_R_Nm = Throttle_Torque-d;
    return;
else
%opposite case
Torque_L_Nm = Throttle_Torque-d;
Torque_R_Nm = Throttle_Torque;
return;
end
end

== matlab function TheBigOne/SKIDPAD/TC+TV/Rigid Axle with TC 2024  ==
  data: MAX_SLR input; Throttle_Torque_R input; Throttle_Torque_L input; Motor_Torque_RR output; Motor_Torque_RL output; el_Vel_X input; Vel_ms_wheel_RR input; Vel_ms_wheel_RL input
function [Motor_Torque_RR, Motor_Torque_RL] = TC_2024(MAX_SLR,Throttle_Torque_R, Throttle_Torque_L, el_Vel_X, Vel_ms_wheel_RR, Vel_ms_wheel_RL)
    persistent correction
    if isempty(correction)
        correction = 0;
    end
if (el_Vel_X < 0.5 || Vel_ms_wheel_RR < 0.5 || Vel_ms_wheel_RL < 0.5)
    correction = 0;
    Motor_Torque_RR = Throttle_Torque_R;
    Motor_Torque_RL = Throttle_Torque_L;
    return;
else

% SLIP RATIO CALCULATIONS
    % calculate slip ratio
    if(el_Vel_X == 0 || Vel_ms_wheel_RR == 0)
        SLR_RR = 1;
    else
    SLR_RR = (Vel_ms_wheel_RR / el_Vel_X);
    end
    if(el_Vel_X == 0 || Vel_ms_wheel_RL == 0)
        SLR_RL = 1;
    else
    SLR_RL = (Vel_ms_wheel_RL / el_Vel_X);
    end


% SLIP RATIO CALCULATIONS
    % calculate slip ratio
    SLR = max(SLR_RR, SLR_RL);

% CHECK FOR EXCESIVE SLIPPING
    % SLIP RATIO LESSER THAN MAXIMUM SLIP RATIO => apply max torque times throttle factor
        if(SLR < MAX_SLR)
            Motor_Torque_RR = Throttle_Torque_R; 
            Motor_Torque_RL = Throttle_Torque_L;
            correction = 0; %set correction to 0 as tyre is not slipping
            return;
        else
        % TYRE SLIPPING => TC INTERVENES
            % LOOK FOR THE PREVIOUS CORRECTION [Nm]
            if (correction == 0) % NOT SLIPPING PREVIOUSLY
                correction = 1; % [INTERVAL TO BE DETERMINED] set the correction to the torque we want to substract
                Motor_Torque_RR = Throttle_Torque_R - (1/33*correction^2+1/33*correction); % substract the correction from the torque to apply
                Motor_Torque_RL = Throttle_Torque_L - (1/33*correction^2+1/33*correction);
                return;
            else % TYRE SLIPPING PREVIOUSLY
                correction = correction + 1; % [INTERVAL TO BE DETERMINED] set the correction to the torque we want to substract + previous corrections
                Motor_Torque_RR = Throttle_Torque_R - (1/33*correction^2+1/33*correction); % substract the correction from the torque to apply
                Motor_Torque_RL = Throttle_Torque_L - (1/33*correction^2+1/33*correction);
                return;
            end
        end
end
end

== matlab function TheBigOne/AUTOX1/TC+TV/MATLAB Function ==
  data: steering_max_angle input; Torque_R_Nm output; Torque_L_Nm output; steering input; steering_deadzone input; Throttle_Torque input
function [Torque_R_Nm, Torque_L_Nm] = TV(steering_max_angle, steering, steering_deadzone, Throttle_Torque)
    if abs(steering) <= steering_deadzone % add steering deadzone (º)
        Torque_L_Nm = Throttle_Torque;
        Torque_R_Nm = Throttle_Torque;
        return;
    end
        d = (abs(steering) - steering_deadzone)/(steering_max_angle - steering_deadzone) * Throttle_Torque; %evaluate delta torque for given steering angle
    if d > Throttle_Torque
         d = Throttle_Torque; %force torque to be positive to avoid balance issues
    end
    if steering < -steering_deadzone %if steering left, apply more torque to the inner motor
        Torque_L_Nm = Throttle_Torque;
        Torque_R_Nm = Throttle_Torque-d;
        return;
    else
        %opposite case
        Torque_L_Nm = Throttle_Torque-d;
        Torque_R_Nm = Throttle_Torque;
        return;
    end
end

== matlab function TheBigOne/SKIDPAD/Torque demanded by the driver ==
  data: Throttle_Torque output; AP input; pedal_sat_down input; pedal_sat_up input; max_torque input
function Throttle_Torque  = TT(AP, pedal_sat_down, pedal_sat_up, max_torque)
    if AP <= pedal_sat_down %establish the lower deadzone for the throttle pedal
        Throttle_Response = 0;

    elseif AP >= pedal_sat_up %establish the higher deadzone for the throttle pedal
        Throttle_Response = 1;

    else
        Throttle_Response = ((AP - pedal_sat_down) / (pedal_sat_up - pedal_sat_down)); %evaluate for given input
    end
    Throttle_Torque = Throttle_Response * max_torque; % set torque to max output times pedal factor
end

== matlab function TheBigOne/AUTOX1/Torque demanded by the driver ==
  data: Throttle_Torque output; AP input; pedal_sat_down input; pedal_sat_up input; max_torque input
function Throttle_Torque  = TT(AP, pedal_sat_down, pedal_sat_up, max_torque)
    if AP <= pedal_sat_down %establish the lower deadzone for the throttle pedal
        Throttle_Response = 0;

    elseif AP >= pedal_sat_up %establish the higher deadzone for the throttle pedal
        Throttle_Response = 1;

    else
        Throttle_Response = ((AP - pedal_sat_down) / (pedal_sat_up - pedal_sat_down)); %evaluate for given input
    end
    Throttle_Torque = Throttle_Response * max_torque; % set torque to max output times pedal factor
end
